simulink model "longitudinal_vehicle_dynamics"  (R2025a)
settings: Solver=VariableStepAuto  StartTime=0.0  StopTime=25  RelTol=1e-3
model workspace (MAT data in the model file):
  C = 0.55
  Re = 0.01
  Rw = 0.33415
  force_scaling = 2000
  m = 1200
  torque_scaling = 2000
  v0 = 20
libraries: SignalEditorBlockLib x1
settings Model: Creator=howardchueh  LastModifiedBy=howardchueh

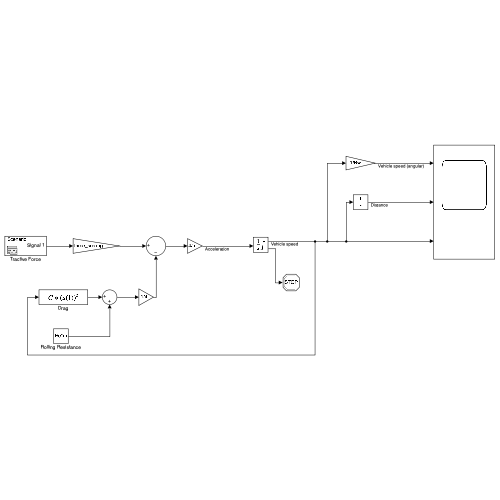
[thumbnail: Simulink's stored preview of the top-level diagram]
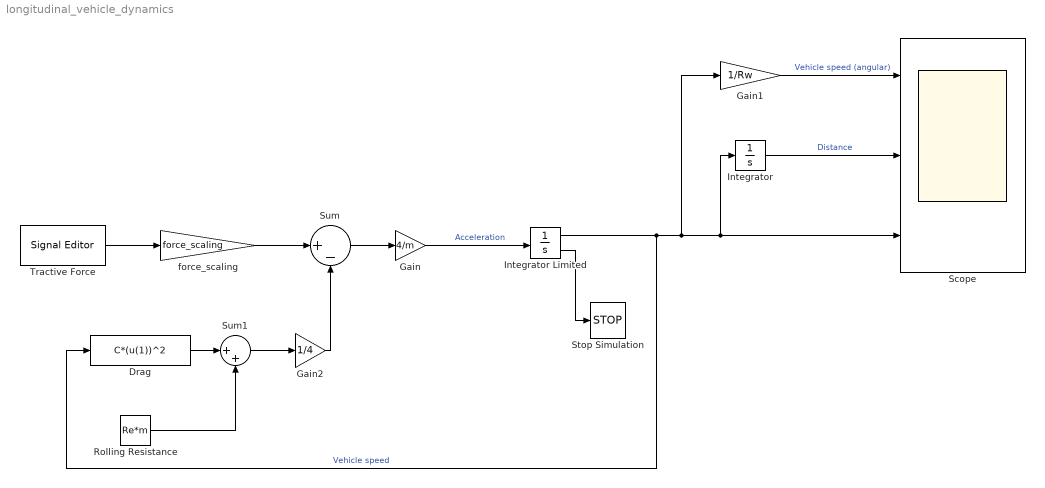
== system longitudinal_vehicle_dynamics ==
  Drag : Fcn  Expr=C*(u(1))^2
  Gain : Gain  Gain=4/m
  Gain1 : Gain  Gain=1/Rw
  Gain2 : Gain  Gain=1/4
  Integrator : Integrator
  Integrator Limited : Integrator  InitialCondition=30  LimitOutput=on  UpperSaturationLimit=100  LowerSaturationLimit=0  ShowSaturationPort=on
  Rolling Resistance : Constant  Value=Re*m
  Scope : Scope  NumInputPorts=3
      settings: ActiveDisplayYMinimum=-19.545046028120741  ActiveDisplayYMaximum=175.90541425308672
  Stop Simulation : Stop
  Sum : Sum  Inputs=|+-
  Sum1 : Sum  Inputs=|++
  Tractive Force : SignalEditorBlockLib/Signal Editor  FileName=tractive_force.mat  ActiveScenario=Scenario  ActiveSignal=Signal 1  IsBus=off  OutputBusObjectStr=Bus: BusObject  SampleTime=0  ZeroCross=off  OutputAfterFinalValue=Setting to zero  Unit=inherit  PreserveSignalName=on  ApplySigPropsToAllScenarios=on  ApplySigPropsToAllSignals=off  SignalPropertySource=Dialog parameters
  force_scaling : Gain  Gain=force_scaling
  wires:
  Tractive Force/1 -> force_scaling/1
  force_scaling/1 -> Sum/1
  Sum/1 -> Gain/1
  Gain2/1 -> Sum/2
  Sum1/1 -> Gain2/1
  Rolling Resistance/1 -> Sum1/2
  Drag/1 -> Sum1/1
  Gain/1 -> Integrator Limited/1  "Acceleration"
  Integrator/1 -> Scope/2  "Distance"
  Gain1/1 -> Scope/1  "Vehicle speed (angular)"
  Integrator Limited/1 -> Drag/1, Gain1/1, Integrator/1, Scope/3  "Vehicle speed"
  Integrator Limited/2 -> Stop Simulation/1
